simulink model "Ctrl_For_HRV_20260625"  (R2024b)
settings: Solver=ode4  StartTime=0.0  StopTime=22  FixedStep=0.02  RelTol=1e-3
InitFcn:
  | Parameter;
values from neighbouring files (symbols this model uses):
  h_alpha = h_1    (= 0.02)    [Parameter.m]
  h_beta = h_1    (= 0.02)    [Parameter.m]
  h_miu = h_1    (= 0.02)    [Parameter.m]
  h_p = h_1    (= 0.02)    [Parameter.m]
  h_q = h_1    (= 0.02)    [Parameter.m]
  h_r = h_1    (= 0.02)    [Parameter.m]
  r_alpha = r_1    (= 0.15)    [Parameter.m]
  r_beta = r_1    (= 0.15)    [Parameter.m]
  r_miu = r_3    (= 0.1)    [Parameter.m]
  r_p = r_2    (= 1.8)    [Parameter.m]
  r_q = r_2    (= 1.8)    [Parameter.m]
  r_r = r_2    (= 1.8)    [Parameter.m]
  xishu = 0    [Parameter.m]
  xishu_D_0 = 0.3    [Parameter.m]
  xishu_L_0 = 0.2    [Parameter.m]
  xishu_l_0 = 0.23    [Parameter.m]
  xishu_m_0 = 0.17    [Parameter.m]
  xishu_n_0 = 0.09    [Parameter.m]
  xishu_Y_0 = 0.14    [Parameter.m]
undefined symbols (not defined in the file or in its folder): CCI_DUI_AngleRate_Controller, CCI_DUI_FlowAngle_Controller, fhan, PNG_2026_6_23
libraries: simulink x12
(part 2 of 2)

== matlab function Ctrl_For_HRV_20260625/MATLAB Function1 ==
  data: u input; y output
function y = fcn(u)

omega_c = [alpha_c;beta_c;miu_c];
dot_omega_c = [dot_alpha_c;dot_beta_c;dot_miu_c];
ddot_omega_c = [ddot_alpha_c;ddot_beta_c;ddot_miu_c];
e_wd = [e_wd_1;e_wd_2;e_wd_3];
dot_e_wd = [dot_e_wd_1;dot_e_wd_2;dot_e_wd_3];

[Ma,Q] = M_Q(H,V);
%计算气动系数
[C_L_alpha,C_L_delta_a,C_L_delta_e] = Coefficient_Lift(alpha,Ma,delta_a,delta_e,delta_r);
[C_D_alpha,C_D_delta_a,C_D_delta_e,C_D_delta_r] = Coefficient_Drag(alpha,Ma,delta_a,delta_e,delta_r);
[C_Y_beta,C_Y_delta_a,C_Y_delta_e,C_Y_delta_r] = Coefficient_Side(alpha,Ma,delta_a,delta_e,delta_r);
% [C_L_alpha,C_L_delta_a,C_L_delta_e] = Coefficient_Lift(alpha,Ma,0,0,0);
% [C_D_alpha,C_D_delta_a,C_D_delta_e,C_D_delta_r] = Coefficient_Drag(alpha,Ma,0,0,0);
% [C_Y_beta,C_Y_delta_a,C_Y_delta_e,C_Y_delta_r] = Coefficient_Side(alpha,Ma,0,0,0);
[C_l_beta,C_l_delta_a,C_l_delta_e,C_l_delta_r,C_l_r,C_l_p] = Coefficient_RollingMoment(alpha,Ma,delta_a,delta_e,delta_r);
[C_m_alpha,C_m_delta_a,C_m_delta_e,C_m_delta_r,C_m_q] = Coefficient_PitchMoment(alpha,Ma,delta_a,delta_e,delta_r);
[C_n_beta,C_n_delta_a,C_n_delta_e,C_n_delta_r,C_n_p,C_n_r] = Coefficient_YawingMoment(alpha,Ma,delta_a,delta_e,delta_r);
C_L = C_L_alpha+C_L_delta_a+C_L_delta_e;
C_D = C_D_alpha+C_D_delta_a+C_D_delta_e+C_D_delta_r;
C_Y = C_Y_beta*beta+C_Y_delta_a+C_Y_delta_e+C_Y_delta_r;
C_l = C_l_beta*beta+C_l_delta_a*delta_a+C_l_delta_e*delta_e+C_l_delta_r*delta_r+C_l_r*(r*b/(2*V))+C_l_p*(p*b/(2*V));
C_m = C_m_alpha+C_m_delta_a*delta_a+C_m_delta_e*delta_e+C_m_delta_r*delta_r+C_m_q*(q*c/(2*V));
C_n = C_n_beta*beta+C_n_delta_a*delta_a+C_n_delta_e*delta_e+C_n_delta_r*delta_r+C_n_p*(p*b/(2*V))+C_n_r*(r*b/(2*V));

%摄动值
Delta_C_L = C_L_d*C_L; Delta_C_D = C_D_d*C_D; Delta_C_Y = C_Y_d*C_Y;
Delta_C_l = C_l_d*C_l; Delta_C_m = C_m_d*C_m; Delta_C_n = C_n_d*C_n;

%%重力加速度
R = earth_r+H; %R为地心距
g = (earth_r/R)^2*g0;

%%
% 模型调整
%先得到系数
Coefficient_C_L_alpha = 1.86e-2 + 1.01e-4 + 1.01e-4;
C_L_else = C_L - Coefficient_C_L_alpha * alpha;

Coefficient_C_Y_alpha = -1.12e-7 + 1.12e-7 + 4.86e-20;
C_Y_else = C_Y - Coefficient_C_Y_alpha * alpha;

Coefficient_C_l_beta_0 = -1.402e-1;
C_l_beta_else = C_l_beta - Coefficient_C_l_beta_0;

Coefficient_C_l_p_0 = -2.99e-1;
C_l_p_else = C_l_p - Coefficient_C_l_p_0;

Coefficient_C_l_r_0 = 3.82e-1;
C_l_r_else = C_l_r - Coefficient_C_l_r_0;

Coefficient_C_m_alpha_alpha = -2.260e-3 -6.59e-5 -6.59e-5;
C_m_alpha_else = C_m_alpha - Coefficient_C_m_alpha_alpha*alpha;

Coefficient_C_m_q_0 = -1.36;
C_m_q_else = C_m_q - Coefficient_C_m_q_0;

Coefficient_C_n_p_0 = 3.68e-1;
C_n_p_else = C_n_p - Coefficient_C_n_p_0;


%将模改写为面向控制的形式
d_alpha = 0.1*0.005*sin(0.2*pi*t); d_beta = 0.1*0.005*sin(0.2*pi*t); d_miu = 0.1*0.005*sin(0.2*pi*t);
d_p = 0.1*0.007*sin(pi*t); d_q = 0.1*0.01*sin(pi*t); d_r = 0;
%姿态角环
omega = [alpha;beta;miu];
w = [p;q;r];
u = [delta_a;delta_e;delta_r];

W_oo = [-Q*S*Coefficient_C_L_alpha,0,0;
        Q*S*Coefficient_C_Y_alpha,0,0;
        Q*S*(Coefficient_C_L_alpha*(tan(theta)*sin(miu)+tan(beta))+Coefficient_C_Y_alpha*tan(theta)*cos(beta)*cos(miu))];
F_else = [-Q*S*C_L_else,0,0;
        Q*S*C_Y_else,0,0;
        Q*S*(C_L_else*(tan(theta)*sin(miu)+tan(beta))+C_Y_else*tan(theta)*cos(beta)*cos(miu))];
f_o = [(m*g*cos(theta)*cos(miu))/(m*V*cos(beta));
       (m*g*cos(theta)*sin(miu))/(m*V);
       (-m*g*cos(theta)*tan(beta)*cos(miu))/(m*V)];
g_o = [-p*cos(alpha)*tan(beta) - r*sin(alpha)*tan(beta);
       p*sin(alpha);
       r*sin(alpha)*sec(beta)];
W_ow = [0,1,0;
        0,0,-cos(alpha);
        cos(alpha)*sec(beta)];
phi_s = [(-Q*S*Delta_C_L)/(m*V*cos(beta))+d_alpha;
         (Q*S*Delta_C_Y)/(m*V)+d_beta;
         (Q*S*Delta_C_L*(tan(theta)*sin(miu)+tan(beta))+Q*S*Delta_C_Y*tan(theta)*cos(beta)*cos(miu))/(m*V)+d_miu];
D_F = f_o + F_else + phi_s;
Dot_o = W_oo*omega + W_ow*w + g_o + D_F;

%角速度环
W_wo = [0,Q*S*b*Coefficient_C_l_beta_0/I_xx,0;
        Q*S*c_A*Coefficient_C_m_alpha_alpha/I_yy,0,0;
        0,0,0];
W_ww = [(Q*S*b/I_xx)*(Coefficient_C_l_p_0*b/(2*V)),0,(Q*S*b/I_xx)*(Coefficient_C_l_r_0*b/(2*V));
        0,(Q*S*c_A/I_yy)*Coefficient_C_m_q_0*c_A/(2*V),0;
        (Q*S*b/I_zz)*Coefficient_C_n_p_0*b/(2*V),0,0];
M_else = [(Q*S*b/I_xx)*(C_l_beta_else*beta+C_l_p_else*(p*b/(2*V))+C_l_r_else*(r*b/(2*V)));
          (Q*S*c_A/I_yy)*(C_m_alpha_else+C_m_q_else*(q*c_A/(2*V)));
          (Q*S*b/I_zz)*(C_n_beta*beta+C_n_p_else*(p*b/(2*V))+C_n_r*(r*b/(2*V)))];
f_w = [(I_yy-I_zz)*q*r/I_xx;
       (I_zz-I_xx)*p*r/I_yy;
       (I_xx-I_yy)*p*q/I_zz];
g_f = [Q*S*b*C_l_delta_a/I_xx   Q*S*b*C_l_delta_e/I_xx   Q*S*b*C_l_delta_r/I_xx;
       Q*S*c_A*C_m_delta_a/I_yy Q*S*c_A*C_m_delta_e/I_yy Q*S*c_A*C_m_delta_r/I_yy;
       Q*S*b*C_n_delta_a/I_zz   Q*S*b*C_n_delta_e/I_zz   Q*S*b*C_n_delta_r/I_zz];
phi_f = [Q*S*b*Delta_C_l/I_xx+d_p;
         Q*S*c_A*Delta_C_m/I_yy+d_q;
         Q*S*b*Delta_C_n/I_zz+d_r];
D_M = M_else + phi_f;

Dot_w = W_ww*w + W_wo*omega + g_f*u + f_w + D_M;
%%
%计算误差系统
%e_omega = omega - omega_c;
%e_w = W_ow*w + W_oo*omega_c - dot_omega_c - e_wd;

A_oo = W_oo;
A_ww = W_ow*W_ww*inv(W_ow);
A_wo = W_ow*W_wo;
B = W_ow*g_f;
h = (W_ow*W_wo - W_ow*W_ww*inv(W_ow)*W_oo)*omega_c + (W_oo+W_ow*W_ww*inv(W_ow))*dot_omega_c - ddot_omega_c;
r = W_ow*W_ww*inv(W_ow)*e_wd - dot_e_wd;
D_M_error = W_ow*D_M;

dot_e_omega = A_oo*e_omega + e_w + e_wd + g_o + D_F;
dot_e_w = A_ww*e_w + A_wo*e_omega + f_w + B*u + h + r + D_M_error;


dot_error_alpha = dot_e_omega(1); dot_error_beta = dot_e_omega(2); dot_error_miu = dot_e_omega(3);
dot_error_w_1 = dot_e_w(1); dot_error_w_2 = dot_e_w(2); dot_error_w_3 = dot_e_w(3);

x_dot=[dot_error_alpha;dot_error_beta;dot_error_miu;dot_error_w_1;dot_error_w_2;dot_error_w_3];
sys = x_dot;



y = u;

== matlab function Ctrl_For_HRV_20260625/PNG/MATLAB Function ==
  data: V input; v output; theta input; psi input
function v = fcn(V,theta,psi)
dot_X = V*cos(theta)*cos(psi);
dot_Y = V*cos(theta)*sin(psi);
dot_H = V*sin(theta);

v=[dot_X;dot_Y;dot_H];

== matlab function Ctrl_For_HRV_20260625/PNG/MATLAB Function1 ==
  data: ny_cmd input; alpha_cmd output; nz_cmd input; miu_cmd output; Q input; H input; Ma input; miu_last input
function [alpha_cmd, miu_cmd] = fcn(ny_cmd, nz_cmd, Q, H, Ma, miu_last)                                                                                                                                     
% Convert overload commands to smooth alpha and bank commands.                                                                                                                                              
S = 334.73; m = 63504; earth_r = 6371000; g0 = 9.8060;                                                                                                                                                      
sampleTime = 0.02; overloadRateLimit = 10.0;                                                                                                                                                                
alphaRateLimit = 10.0; bankRateLimit = 30.0*pi/180; commandTau = 0.25;                                                                                                                                      
g = (earth_r/(earth_r + H))^2*g0;                                                                                                                                                                           
persistent nyState nzState alphaState initialized                                                                                                                                                           
if isempty(initialized)                                                                                                                                                                                     
nyState = ny_cmd; nzState = nz_cmd; alphaState = 0.0; initialized = true;                                                                                                                               
end                                                                                                                                                                                                         
nyLimited = rateLimit(ny_cmd, nyState, overloadRateLimit, sampleTime);                                                                                                                                      
nzLimited = rateLimit(nz_cmd, nzState, overloadRateLimit, sampleTime);                                                                                                                                      
blend = sampleTime/(commandTau + sampleTime);                                                                                                                                                               
nyState = nyState + blend*(nyLimited - nyState);                                                                                                                                                            
nzState = nzState + blend*(nzLimited - nzState);                                                                                                                                                            
ny = nyState; nz = nzState;                                                                                                                                                                                 
nL = hypot(ny, nz);                                                                                                                                                                                         
if nL < 1e-4                                                                                                                                                                                                
miu_raw = miu_last;                                                                                                                                                                                     
else                                                                                                                                                                                                        
miu_raw = atan2(ny, nz);                                                                                                                                                                                
end                                                                                                                                                                                                         
miu_target = miu_last + wrapToPiLocal(miu_raw - miu_last);                                                                                                                                                  
miu_cmd = miu_last + rateLimit(miu_target - miu_last, 0.0, bankRateLimit, sampleTime);                                                                                                                      
miu_cmd = wrapToPiLocal(miu_cmd);                                                                                                                                                                           
alpha_min = -30; alpha_max = 30;                                                                                                                                                                            
CL_min = CL_of_alpha(alpha_min, Ma); CL_max = CL_of_alpha(alpha_max, Ma);                                                                                                                                   
CL_cmd = nL*m*g/max(Q*S, 1e-6);                                                                                                                                                                             
CL_cmd = min(max(CL_cmd, min(CL_min, CL_max)), max(CL_min, CL_max));                                                                                                                                        
alphaRaw = solveAlpha(CL_cmd, alpha_min, alpha_max, Ma);                                                                                                                                                    
if alphaState < alpha_min || alphaState > alpha_max                                                                                                                                                         
alphaState = alphaRaw;                                                                                                                                                                                  
end                                                                                                                                                                                                         
alphaLimited = rateLimit(alphaRaw, alphaState, alphaRateLimit, sampleTime);                                                                                                                                 
alphaState = alphaState + blend*(alphaLimited - alphaState);                                                                                                                                                
alpha_cmd = saturate(alphaState, alpha_min, alpha_max);                                                                                                                                                     
end                                                                                                                                                                                                         
function alpha = solveAlpha(CL_cmd, alpha_min, alpha_max, Ma)                                                                                                                                               
alpha = alpha_min; bestErr = abs(CL_of_alpha(alpha_min, Ma) - CL_cmd);                                                                                                                                  
for k = 1:120                                                                                                                                                                                           
a = alpha_min + (alpha_max - alpha_min)*k/120;                                                                                                                                                      
err = abs(CL_of_alpha(a, Ma) - CL_cmd);                                                                                                                                                             
if err < bestErr                                                                                                                                                                                    
bestErr = err; alpha = a;                                                                                                                                                                       
end                                                                                                                                                                                                 
end                                                                                                                                                                                                     
end                                                                                                                                                                                                         
function CL = CL_of_alpha(alpha_deg, Ma)                                                                                                                                                                    
CL = (-8.19e-2)+(4.7e-2)*Ma+(1.86e-2)*alpha_deg-(4.73e-4)*(alpha_deg*Ma)-(9.19e-3)*Ma^2-(1.52e-4)*alpha_deg^2+(5.99e-7)*(alpha_deg*Ma)^2+(7.74e-4)*Ma^3+(4.08e-6)*alpha_deg^3-(2.93e-5)*Ma^4+(4.12e-7)*Ma^5;
end                                                                                                                                                                                                         
function y = rateLimit(u, yPrev, rateLimitValue, sampleTime)                                                                                                                                                
maxStep = rateLimitValue*sampleTime;                                                                                                                                                                        
y = yPrev + min(max(u - yPrev, -maxStep), maxStep);                                                                                                                                                         
end                                                                                                                                                                                                         
function y = saturate(x, lo, hi)                                                                                                                                                                            
y = min(max(x, lo), hi);                                                                                                                                                                                    
end                                                                                                                                                                                                         
function ang = wrapToPiLocal(ang)                                                                                                                                                                           
ang = mod(ang + pi, 2*pi) - pi;                                                                                                                                                                             
end

== matlab function Ctrl_For_HRV_20260625/PNG/MATLAB Function2 ==
  data: V input; f_psi output; theta input; psi input; lat input; H input
function f_psi = earth_rotation(V,theta,psi,lat,H)

earth_r = 6371000;
w_e = 7.292116000000000e-05;
R = earth_r + H;
f_psi = V*cos(theta)*sin(psi)*tan(lat)/R ...
      + 2*w_e*(sin(lat)-cos(lat)*cos(psi)*tan(theta)) ...
      + w_e^2*R*cos(lat)*sin(lat)*sin(psi)/(V*cos(theta));

== matlab function Ctrl_For_HRV_20260625/MATLAB Function2 ==
  data: ny output; nz output; position_t input; vt input; hgv_states input; theta_f input; kai_f input
function [ny, nz] = Prop_guidance(position_t, vt, hgv_states, theta_f, kai_f)
% Smooth moving-aimpoint PN with terminal flight-path-angle constraint.
H = hgv_states(1); lat = hgv_states(3); V = max(hgv_states(4),1.0);
theta = hgv_states(5); psi = hgv_states(6);
X = hgv_states(7); alt = hgv_states(8); Y = hgv_states(9);
thetaDesired = theta_f*pi/180; psiDesired = kai_f*pi/180;
vTerminal = [cos(thetaDesired)*cos(psiDesired); ...
    cos(thetaDesired)*sin(psiDesired);sin(thetaDesired)];
rTrue = [position_t(1)-X;position_t(2)-Y;position_t(3)-alt];
realRange = max(norm(rTrue),1.0);
blend = smoothStep((realRange-250.0)/(1500.0-250.0));
leadDistance = min(1000.0,0.02*realRange)*blend;
aimpoint = position_t-leadDistance*vTerminal;
rx = aimpoint(1)-X; ry = aimpoint(2)-Y; rh = aimpoint(3)-alt;
vx = V*cos(theta)*cos(psi);vy = V*cos(theta)*sin(psi);vh = V*sin(theta);
vrx = vt(1)-vx;vry = vt(2)-vy;vrh = vt(3)-vh;
range = max(sqrt(rx^2+ry^2+rh^2),1.0);
closing = max(-(rx*vrx+ry*vry+rh*vrh)/range,50.0);
qTheta = atan2(rh,hypot(rx,ry));qPsi = atan2(ry,rx);
rho2 = max(rx^2+ry^2,1.0);qPsiDot = (rx*vry-ry*vrx)/rho2;
rhoriz = sqrt(rho2);rhorizDot = (rx*vrx+ry*vry)/rhoriz;
qThetaDot = (rhoriz*vrh-rh*rhorizDot)/max(rho2+rh^2,1.0);
thetaErr = wrapToPiLocal(qTheta-theta);psiErr = wrapToPiLocal(qPsi-psi);
tgo = min(max(range/closing,1.0),80.0);
Ntheta = 4.0;Npsi = 4.0;Ktheta = 0.8;Kpsi = 0.8;KterminalTheta = 1.2;KterminalPsi = 1.0;
terminalThetaErr = wrapToPiLocal(thetaDesired-theta);
aTheta = Ntheta*closing*qThetaDot+Ktheta*V*thetaErr/tgo ...
    +KterminalTheta*V*terminalThetaErr/tgo;
terminalPsiErr = wrapToPiLocal(psiDesired-psi);
aPsi = Npsi*closing*qPsiDot+Kpsi*V*cos(theta)*psiErr/tgo ...
    +KterminalPsi*V*cos(theta)*terminalPsiErr/tgo;
g = gravityLocal(H);earth_r = 6371000;omega = 7.292116e-5;R = earth_r+H;
geomTheta = V*cos(theta)/R+2*omega*cos(lat)*sin(psi) ...
    +omega^2*R*cos(lat)*(cos(theta)*cos(lat)+sin(theta)*cos(psi)*sin(lat))/V;
geomPsi = V*cos(theta)*sin(psi)*tan(lat)/R ...
    +2*omega*(sin(lat)-cos(lat)*cos(psi)*tan(theta)) ...
    +omega^2*R*cos(lat)*sin(lat)*sin(psi)/max(V*cos(theta),1.0);
ny = saturate(aTheta/g+cos(theta)-(V/g)*geomTheta,-20.0,20.0);
nz = saturate(aPsi/g-(V*cos(theta)/g)*geomPsi,-20.0,20.0);
end
function y = smoothStep(x)
x = min(max(x,0.0),1.0);y = x*x*(3.0-2.0*x);
end
function y = saturate(x,lo,hi)
y = min(max(x,lo),hi);
end
function ang = wrapToPiLocal(ang)
ang = mod(ang+pi,2*pi)-pi;
end
function g = gravityLocal(H)
earth_r = 6371000;g0 = 9.806;g = (earth_r/(earth_r+H))^2*g0;
end
